simulink model "motor_sim"  (R2023a)
settings: Solver=VariableStepAuto  StartTime=0.0  StopTime=10.0  RelTol=1e-3
values from neighbouring files (symbols this model uses):
  Bm = 10^(-5)    (= 1e-05)    [parameter.m]
  Jm = 3*10^(-5)    (= 3e-05)    [parameter.m]
  Km = 0.0267    [parameter.m]
  L = 5*10^(-3)    (= 0.005)    [parameter.m]
  R = 4    [parameter.m]
settings Model: Creator=USER  LastModifiedBy=USER

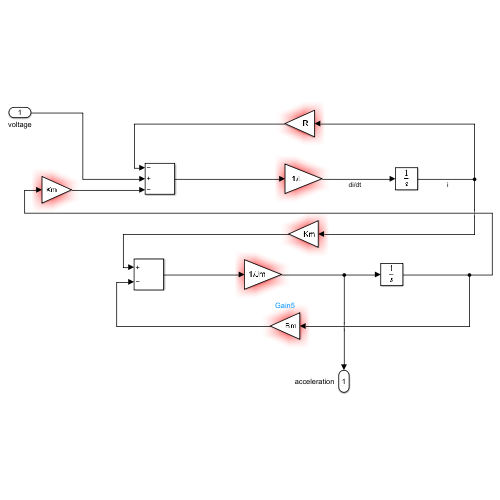
[thumbnail: Simulink's stored preview of the top-level diagram]
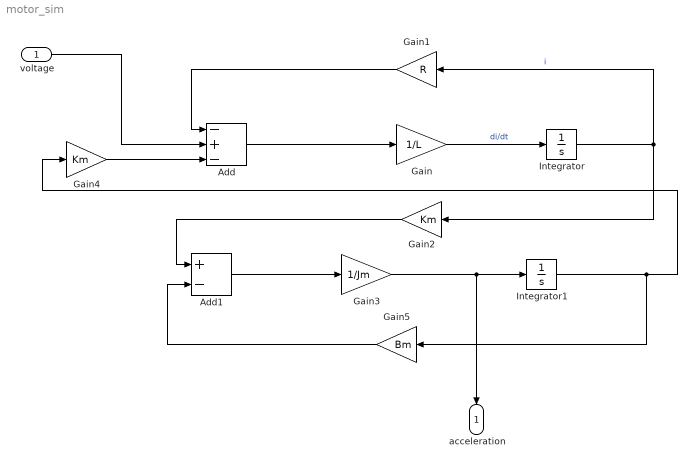
== system motor_sim ==
  voltage : Inport
  Add : Sum  Inputs=-+-
  Add1 : Sum  Inputs=+-
  Gain : Gain  Gain=1/L
  Gain1 : Gain  Gain=R
  Gain2 : Gain  Gain=Km
  Gain3 : Gain  Gain=1/Jm
  Gain4 : Gain  Gain=Km
  Gain5 : Gain  Gain=Bm
  Integrator : Integrator
  Integrator1 : Integrator
  acceleration : Outport
  wires:
  Add/1 -> Gain/1
  Gain/1 -> Integrator/1  "di/dt"
  Integrator/1 -> Gain2/1, Gain1/1  "i"
  Gain1/1 -> Add/1
  voltage/1 -> Add/2
  Add1/1 -> Gain3/1
  Gain3/1 -> acceleration/1, Integrator1/1
  Integrator1/1 -> Gain5/1, Gain4/1
  Gain4/1 -> Add/3
  Gain5/1 -> Add1/2
  Gain2/1 -> Add1/1
